simulink model "SimplePendulum"  (R2014a)
settings: Solver=ode45  StartTime=0.0  StopTime=T  RelTol=1e-3
undefined symbols (not defined in the file): a1, a2, b2, ct, st, tau, thetaBar, x10, x20
settings Model: Creator=mauricio  LastModifiedBy=mauricio
settings DataIOCC: SignalLoggingSaveFormat=ModelDataLogs
settings OptimizationCC: ExpressionDepthLimit=2147483647
settings DebuggingCC: UnderspecifiedInitializationDetection=Classic  SolverPrmCheckMsg=none  FcnCallInpInsideContextMsg=UseLocalSettings  StateNameClashWarn=warning
settings GRTTargetCC: CombineOutputUpdateFcns=off  GRTInterface=on

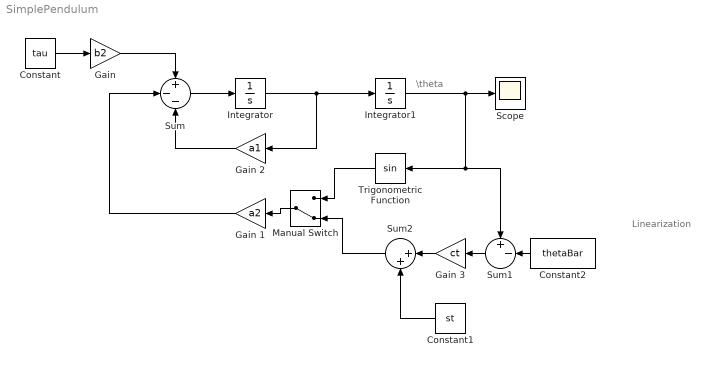
== system SimplePendulum ==
  note: Linearization
  note: \theta
  Constant : Constant  Value=tau
  Constant1 : Constant  Value=st
  Constant2 : Constant  Value=thetaBar
  Gain : Gain  Gain=b2
  Gain 1 : Gain  Gain=a2
  Gain 2 : Gain  Gain=a1
  Gain 3 : Gain  Gain=ct
  Integrator : Integrator  InitialCondition=x10
  Integrator1 : Integrator  InitialCondition=x20
  Manual Switch : ManualSwitch  CurrentSetting=0
  Scope : Scope
      settings: YMin=-3.141592653589793  YMax=3.141592653589793
  Sum : Sum  Inputs=+--
  Sum1 : Sum  Inputs=+-|
  Sum2 : Sum  Inputs=|++
  Trigonometric Function : Trigonometry
  wires:
  Integrator/1 -> Integrator1/1, Gain 2/1
  Integrator1/1 -> Scope/1, Sum1/1, Trigonometric Function/1
  Sum/1 -> Integrator/1
  Constant/1 -> Gain/1
  Gain 2/1 -> Sum/3
  Gain 1/1 -> Sum/2
  Gain/1 -> Sum/1
  Trigonometric Function/1 -> Manual Switch/1
  Manual Switch/1 -> Gain 1/1
  Constant2/1 -> Sum1/2
  Sum1/1 -> Gain 3/1
  Sum2/1 -> Manual Switch/2
  Gain 3/1 -> Sum2/1
  Constant1/1 -> Sum2/2
